simulink subsystem "Aerodynamics_Subsystem"  (R2026a)
settings: Solver=VariableStepAuto
settings Model: Creator=Eeman Aleem  LastModifiedBy=Eeman Aleem

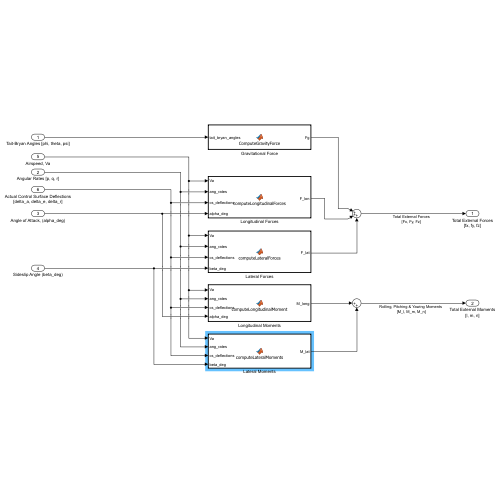
[thumbnail: Simulink's stored preview of the top-level diagram]
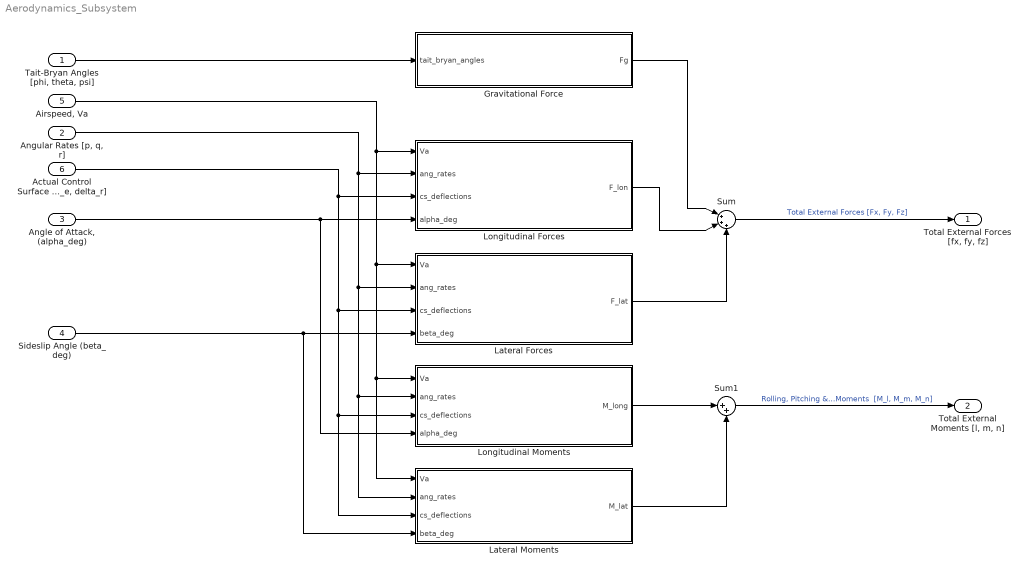
== system Aerodynamics_Subsystem ==
  "Tait-Bryan Angles [phi, theta, psi]" : Inport
  "Angular Rates [p, q, r]" : Inport  Port=2
  "Angle of Attack, (alpha_deg)" : Inport  Port=3
  Sideslip Angle (beta_deg) : Inport  Port=4
  "Airspeed, Va" : Inport  Port=5
  "Actual Control Surface Deflections [delta_a, delta_e, delta_r]" : Inport  Port=6
  Gravitational Force : MATLAB Function  TreatAsAtomicUnit=on
  Lateral Forces : MATLAB Function  TreatAsAtomicUnit=on
  Lateral Moments : MATLAB Function  TreatAsAtomicUnit=on
  Longitudinal Forces : MATLAB Function  TreatAsAtomicUnit=on
  Longitudinal Moments : MATLAB Function  TreatAsAtomicUnit=on
  Sum : Sum  Inputs=|+++
  Sum1 : Sum  Inputs=|++
  "Total External Forces [fx, fy, fz]" : Outport
  "Total External Moments [l, m, n]" : Outport  Port=2
  wires:
  Sum1/1 -> "Total External Moments [l, m, n]"/1  "Rolling, Pitching & Yawing Moments  [M_l, M_m, M_n]"
  Sideslip Angle (beta_deg)/1 -> Lateral Moments/4(beta_deg), Lateral Forces/4(beta_deg)
  Gravitational Force/1(Fg) -> Sum/1
  Lateral Forces/1(F_lat) -> Sum/3
  Lateral Moments/1(M_lat) -> Sum1/2
  Sum/1 -> "Total External Forces [fx, fy, fz]"/1  "Total External Forces [Fx, Fy, Fz]"
  "Tait-Bryan Angles [phi, theta, psi]"/1 -> Gravitational Force/1(tait_bryan_angles)
  Longitudinal Forces/1(F_lon) -> Sum/2
  Longitudinal Moments/1(M_long) -> Sum1/1
  "Actual Control Surface Deflections [delta_a, delta_e, delta_r]"/1 -> Lateral Moments/3(cs_deflections), Longitudinal Moments/3(cs_deflections), Lateral Forces/3(cs_deflections), Longitudinal Forces/3(cs_deflections)
  "Airspeed, Va"/1 -> Lateral Moments/1(Va), Longitudinal Moments/1(Va), Lateral Forces/1(Va), Longitudinal Forces/1(Va)
  "Angular Rates [p, q, r]"/1 -> Lateral Moments/2(ang_rates), Longitudinal Moments/2(ang_rates), Lateral Forces/2(ang_rates), Longitudinal Forces/2(ang_rates)
  "Angle of Attack, (alpha_deg)"/1 -> Longitudinal Moments/4(alpha_deg), Longitudinal Forces/4(alpha_deg)

== matlab function Aerodynamics_Subsystem/Gravitational Force ==
  data: Fg output; tait_bryan_angles input
function Fg = compGravF(tait_bryan_angles)
phi = tait_bryan_angles(1);
theta = tait_bryan_angles(2);
g = GeoConsts.g;
m = GeoConsts.m_full;
% Body-frame gravity force components
Fg = m * g * [-sin(theta);
                 cos(theta)*sin(phi);
                 cos(theta)*cos(phi)];
end

== matlab function Aerodynamics_Subsystem/Longitudinal Forces ==
  data: Va input; ang_rates input; cs_deflections input; F_lon output; alpha_deg input
function F_lon = compLongF(Va, ang_rates, cs_deflections, alpha_deg)
    alpha = deg2rad(alpha_deg);
    delta_e = deg2rad(cs_deflections(2));
    q = ang_rates(2);

    S = GeoConsts.S;
    c = GeoConsts.c;
    AR = GeoConsts.AR;

    Q = 0.5 * 1.225 * Va^2;

    % Stall model
    M = 50;
    alpha0 = 0.47;
    CL_alpha = (pi * AR) / (1 + sqrt(1 + (AR/2)^2));
    sig = (1 + exp(-M*(alpha - alpha0)) + exp(M*(alpha + alpha0))) / ...
          ((1 + exp(-M*(alpha - alpha0))) * (1 + exp(M*(alpha + alpha0))));
    CL_lin = LongitudinalCoeffs.CL0 + CL_alpha * alpha;
    CL_nl  = 2 * sin(alpha) * sin(alpha)^2 * cos(alpha);
    CL = (1 - sig) * CL_lin + sig * CL_nl + ...
         LongitudinalCoeffs.CL_q * (c/(2*Va)) * q + ...
         LongitudinalCoeffs.CL_de * delta_e;

    CD_ind = (CL_lin^2) / (pi * 0.9 * AR);  % e_os = 0.9
    CD = LongitudinalCoeffs.CDp + CD_ind + ...
         LongitudinalCoeffs.CD_q * (c/(2*Va)) * q + ...
         LongitudinalCoeffs.CD_de * abs(delta_e);

    F_lift = Q * S * CL;
    F_drag = Q * S * CD;

    % Convert to body frame
    Fx = -F_drag * cos(alpha) + (-F_lift) * sin(alpha);
    Fz = -F_drag * sin(alpha) - F_lift * cos(alpha);

    F_lon = [Fx; 0; Fz];
end

== matlab function Aerodynamics_Subsystem/Longitudinal Moments ==
  data: Va input; ang_rates input; cs_deflections input; M_long output; alpha_deg input
function M_long = compLongM(Va, ang_rates, cs_deflections, alpha_deg)

    alpha = deg2rad(alpha_deg);
    q = ang_rates(2);
    delta_e = deg2rad(cs_deflections(2));

    if Va < 1e-3
        Va = 1e-3;
    end

    S = GeoConsts.S;
    c = GeoConsts.c;
    rho = 1.225;

    Q = 0.5 * rho * Va^2;

    Cm = LongitudinalCoeffs.Cm0 + ...
         LongitudinalCoeffs.Cm_alpha * alpha + ...
         LongitudinalCoeffs.Cm_q * (c/(2*Va)) * q + ...
         LongitudinalCoeffs.Cm_de * delta_e;

    My = Q * S * c * Cm;

    M_long = [0; My; 0];
end

== matlab function Aerodynamics_Subsystem/Lateral Forces ==
  data: Va input; ang_rates input; cs_deflections input; F_lat output; beta_deg input
function F_lat = compLateralF(Va, ang_rates, cs_deflections, beta_deg)
    beta = deg2rad(beta_deg);
    p = ang_rates(1);
    r = ang_rates(3);
    delta_a = deg2rad(cs_deflections(1));
    delta_r = deg2rad(cs_deflections(3));

    S = GeoConsts.S;
    b = GeoConsts.b;
    Q = 0.5 * 1.225 * Va^2;

    CY = LateralCoeffs.CY0 + ...
         LateralCoeffs.CY_beta * beta + ...
         LateralCoeffs.CY_p * (b/(2*Va)) * p + ...
         LateralCoeffs.CY_r * (b/(2*Va)) * r + ...
         LateralCoeffs.CY_da * delta_a + ...
         LateralCoeffs.CY_dr * delta_r;

    Fy = Q * S * CY;
    F_lat = [0; Fy; 0];
end

== matlab function Aerodynamics_Subsystem/Lateral Moments ==
  data: Va input; ang_rates input; cs_deflections input; M_lat output; beta_deg input
function M_lat = compLateralM(Va, ang_rates, cs_deflections, beta_deg)

    beta = deg2rad(beta_deg);
    p = ang_rates(1);
    r = ang_rates(3);
    delta_a = deg2rad(cs_deflections(1));
    delta_r = deg2rad(cs_deflections(3));

    if Va < 1e-3
        Va = 1e-3;
    end

    S = GeoConsts.S;
    b = GeoConsts.b;
    rho = 1.225;

    Q = 0.5 * rho * Va^2;

    Cl = LateralCoeffs.Cl0 + ...
         LateralCoeffs.Cl_beta * beta + ...
         LateralCoeffs.Cl_p * (b/(2*Va)) * p + ...
         LateralCoeffs.Cl_r * (b/(2*Va)) * r + ...
         LateralCoeffs.Cl_da * delta_a + ...
         LateralCoeffs.Cl_dr * delta_r;

    Cn = LateralCoeffs.Cn0 + ...
         LateralCoeffs.Cn_beta * beta + ...
         LateralCoeffs.Cn_p * (b/(2*Va)) * p + ...
         LateralCoeffs.Cn_r * (b/(2*Va)) * r + ...
         LateralCoeffs.Cn_da * delta_a + ...
         LateralCoeffs.Cn_dr * delta_r;

    Mx = Q * S * b * Cl;
    Mz = Q * S * b * Cn;

    M_lat = [Mx;
             0;
             Mz];
end
